simulink model "MEEN432_Project2_test"  (R2023b)
settings: Solver=VariableStepAuto  StartTime=0.0  StopTime=350  RelTol=1e-3
values from neighbouring files (symbols this model uses):
  alpha_max = 8 * pi/180    (= 0.13962634016)    [MEEN432_Project2_init.m]
  Calpha_f = 40000    [MEEN432_Project2_init.m]
  Calpha_r = 40000    [MEEN432_Project2_init.m]
  inertia = 1600    [MEEN432_Project2_init.m]
  lf = 1.5    [MEEN432_Project2_init.m]
  lr = 1.0    (= 1)    [MEEN432_Project2_init.m]
  mass = 1000    [MEEN432_Project2_init.m]
  omega0 = 0    [MEEN432_Project2_init.m]
  psi0 = 0    [MEEN432_Project2_init.m]
  vd = 10    [MEEN432_Project2_init.m]
  vx_max = 0.1    [MEEN432_Project2_init.m]
  vy0 = 0    [MEEN432_Project2_init.m]
  x_track = [x1 , R*cos(t1) + L , x2, R*cos(t2)]    [MEEN432_Project2_init.m]
  y_track = [y1, R*sin(t1) + R , y2 , R*sin(t2) + R]    [MEEN432_Project2_init.m]
settings Model: Creator=flare  LastModifiedBy=flare

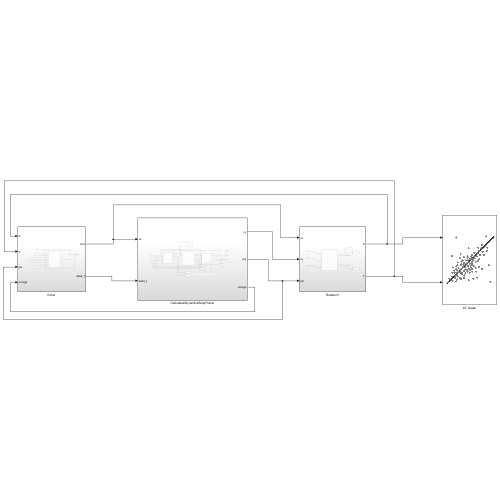
[thumbnail: Simulink's stored preview of the top-level diagram]
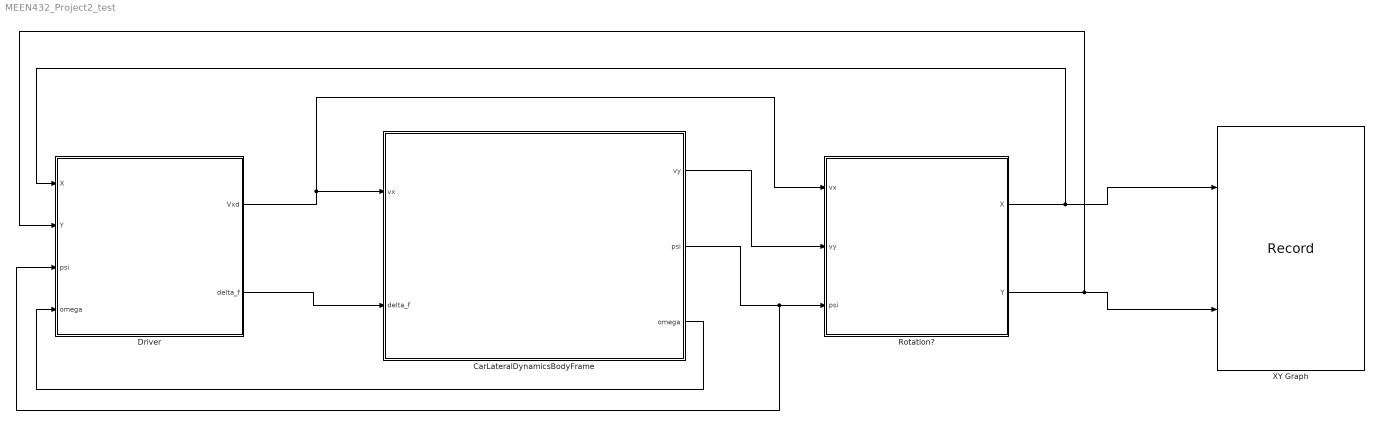
== system MEEN432_Project2_test ==
  CarLateralDynamicsBodyFrame : Subsystem
  Driver : Subsystem
  Rotation? : Subsystem
  XY Graph : Record  FileSettingsInternal="{\"entries\":[{\"content\":{\"excelSettings\":{\"content\":{},\"type\":\"Streamout.ExcelSettings\"}},\"type\":\"Streamout.FileSettingStorage\",\"uuid\":\"\"}],\"packageUris\":[\"http:\\/\\/schema.mathworks.com\\/mf0\\/streamout_blocks\\/R2020a\"],\"version\":\"1.0\"}"  Layout=[1 1]  SignalsInternal="{\"entries\":[{\"content\":{\"signals\":[{\"content\":{\"blockPath\":[],\"dimensions\":[1],\"domain\":\"\",\"lineColor\":\"#139fff\",\"plots\":[1],\"port\":1,\"sid\":[\"\"],\"signalID\":693,\"signalName\":\"Rotation?:1\"},\"type\":\"RecordBlkView.Signal\",\"uuid\":\"\"},{\"content\":{\"blockPath\":[],\"dimensions\":[1],\"domain\":\"\",\"lineColor\":\"#ff6929\",\"plots\":[1],\"port\":2,\"sid\":[\"\"],\"signalID\":697,\"signalName\":\"Rotation?:2\"},\"type\":\"RecordBlkView.Signal\",\"uuid\":\"\"}]},\"type\":\"RecordBlkView.InputSignals\",\"uuid\":\"\"}],\"packageUris\":[\"http:\\/\\/schema.mathworks.com\\/mf0\\/streamout_blocks\\/R2020a\"],\"version\":\"1.0\"}"  VisualizationBindings="{\"xyplotplugin\":{\"info\":[{\"series\":[{\"bindingParametersList\":[{\"parameter\":\"X-Axis\",\"signalID\":693,\"signalName\":\"Rotation?:1\"},{\"parameter\":\"Y-Axis\",\"signalID\":697,\"signalName\":\"Rotation?:2\"}],\"seriesID\":48390}],\"subplotID\":1}]}}"  CompatibilityTag=XY
  wires:
  Rotation?/1(X) -> Driver/1(X), XY Graph/1
  Rotation?/2(Y) -> Driver/2(Y), XY Graph/2
  Driver/1(Vxd) -> Rotation?/1(vx), CarLateralDynamicsBodyFrame/1(vx)
  Driver/2(delta_f) -> CarLateralDynamicsBodyFrame/2(delta_f)
  CarLateralDynamicsBodyFrame/1(vy) -> Rotation?/2(vy)
  CarLateralDynamicsBodyFrame/2(psi) -> Driver/3(psi), Rotation?/3(psi)
  CarLateralDynamicsBodyFrame/3(omega) -> Driver/4(omega)

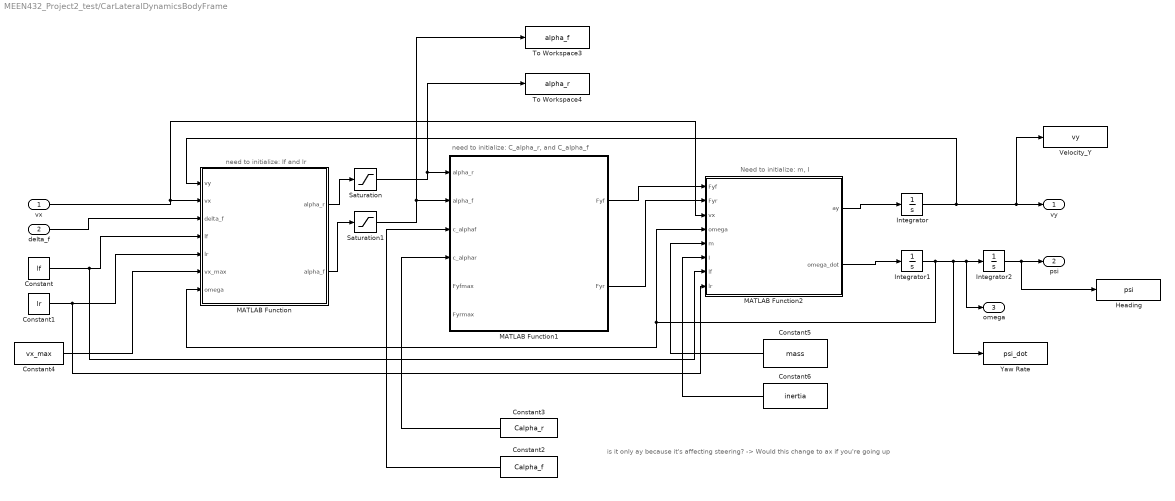
== system MEEN432_Project2_test/CarLateralDynamicsBodyFrame ==
  note: need to initialize: lf and lr
  note: need to initialize: C_alpha_r, and C_alpha_f
  note: is it only ay because it's affecting steering? -> Would this change to ax if you're going up
  note: Need to initialize: m, I
  vx : Inport
  delta_f : Inport  Port=2
  Constant : Constant  Value=lf
  Constant1 : Constant  Value=lr
  Constant2 : Constant  Value=Calpha_f
  Constant3 : Constant  Value=Calpha_r
  Constant4 : Constant  Value=vx_max
  Constant5 : Constant  Value=mass
  Constant6 : Constant  Value=inertia
  Heading : ToWorkspace  VariableName=psi  SaveFormat=Timeseries  SampleTime=-1
  Integrator : Integrator  InitialCondition=vy0
  Integrator1 : Integrator  InitialCondition=omega0
  Integrator2 : Integrator  InitialCondition=psi0
  MATLAB Function : MATLAB Function  TreatAsAtomicUnit=on
  MATLAB Function1 : MATLAB Function  TreatAsAtomicUnit=on
  MATLAB Function2 : MATLAB Function  TreatAsAtomicUnit=on
  Saturation : Saturate  UpperLimit=alpha_max
  Saturation1 : Saturate  UpperLimit=alpha_max
  To Workspace3 : ToWorkspace  VariableName=alpha_f  SaveFormat=Timeseries  SampleTime=-1
  To Workspace4 : ToWorkspace  VariableName=alpha_r  SaveFormat=Timeseries  SampleTime=-1
  Velocity_Y : ToWorkspace  VariableName=vy  SaveFormat=Timeseries  SampleTime=-1
  Yaw Rate : ToWorkspace  VariableName=psi_dot  SaveFormat=Timeseries  SampleTime=-1
  vy : Outport
  psi : Outport  Port=2
  omega : Outport  Port=3
  wires:
  MATLAB Function/1(alpha_r) -> Saturation/1
  MATLAB Function/2(alpha_f) -> Saturation1/1
  MATLAB Function2/2(omega_dot) -> Integrator1/1
  MATLAB Function2/1(ay) -> Integrator/1
  Integrator1/1 -> MATLAB Function2/4(omega), MATLAB Function/7(omega), Yaw Rate/1, omega/1, Integrator2/1
  Integrator/1 -> MATLAB Function/1(vy), Velocity_Y/1, vy/1
  Integrator2/1 -> Heading/1, psi/1
  vx/1 -> MATLAB Function2/3(vx), MATLAB Function/2(vx)
  delta_f/1 -> MATLAB Function/3(delta_f)
  Saturation/1 -> To Workspace4/1, MATLAB Function1/1(alpha_r)
  Saturation1/1 -> To Workspace3/1, MATLAB Function1/2(alpha_f)
  MATLAB Function1/1(Fyf) -> MATLAB Function2/1(Fyf)
  MATLAB Function1/2(Fyr) -> MATLAB Function2/2(Fyr)
  Constant/1 -> MATLAB Function2/7(lf), MATLAB Function/4(lf)
  Constant1/1 -> MATLAB Function2/8(lr), MATLAB Function/5(lr)
  Constant2/1 -> MATLAB Function1/3(c_alphaf)
  Constant3/1 -> MATLAB Function1/4(c_alphar)
  Constant4/1 -> MATLAB Function/6(vx_max)
  Constant5/1 -> MATLAB Function2/5(m)
  Constant6/1 -> MATLAB Function2/6(I)

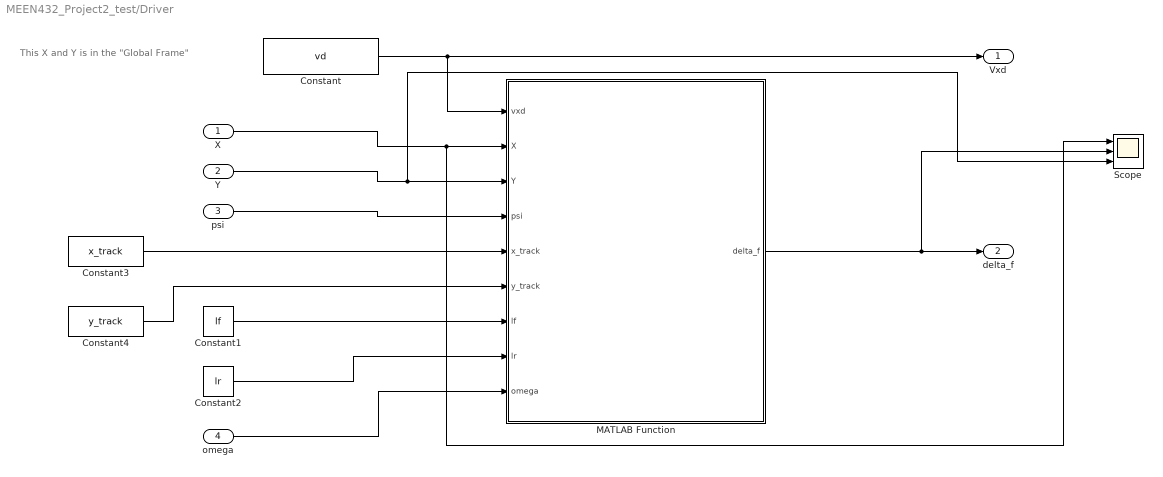
== system MEEN432_Project2_test/Driver ==
  note: This X and Y is in the "Global Frame"
  X : Inport
  Y : Inport  Port=2
  psi : Inport  Port=3
  omega : Inport  Port=4
  Constant : Constant  Value=vd
  Constant1 : Constant  Value=lf
  Constant2 : Constant  Value=lr
  Constant3 : Constant  Value=x_track  VectorParams1D=off
  Constant4 : Constant  Value=y_track  VectorParams1D=off
  MATLAB Function : MATLAB Function  TreatAsAtomicUnit=on
  Scope : Scope  NumInputPorts=3
  Vxd : Outport
  delta_f : Outport  Port=2
  wires:
  Y/1 -> Scope/3, MATLAB Function/3(Y)
  psi/1 -> MATLAB Function/4(psi)
  omega/1 -> MATLAB Function/9(omega)
  MATLAB Function/1(delta_f) -> Scope/2, delta_f/1
  X/1 -> Scope/1, MATLAB Function/2(X)
  Constant1/1 -> MATLAB Function/7(lf)
  Constant2/1 -> MATLAB Function/8(lr)
  Constant/1 -> MATLAB Function/1(vxd), Vxd/1
  Constant3/1 -> MATLAB Function/5(x_track)
  Constant4/1 -> MATLAB Function/6(y_track)

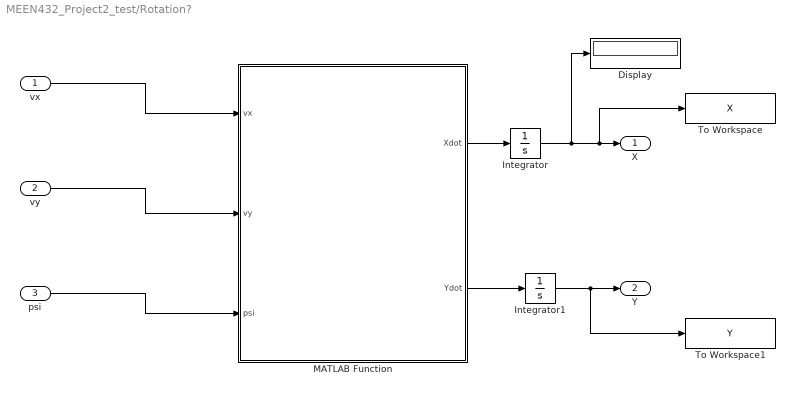
== system MEEN432_Project2_test/Rotation? ==
  vx : Inport
  vy : Inport  Port=2
  psi : Inport  Port=3
  Display : Display
  Integrator : Integrator
  Integrator1 : Integrator
  MATLAB Function : MATLAB Function  TreatAsAtomicUnit=on
  To Workspace : ToWorkspace  VariableName=X  SaveFormat=Timeseries  SampleTime=-1
  To Workspace1 : ToWorkspace  VariableName=Y  SaveFormat=Timeseries  SampleTime=-1
  X : Outport
  Y : Outport  Port=2
  wires:
  vx/1 -> MATLAB Function/1(vx)
  vy/1 -> MATLAB Function/2(vy)
  MATLAB Function/2(Ydot) -> Integrator1/1
  Integrator1/1 -> To Workspace1/1, Y/1
  psi/1 -> MATLAB Function/3(psi)
  MATLAB Function/1(Xdot) -> Integrator/1
  Integrator/1 -> Display/1, To Workspace/1, X/1

== matlab function MEEN432_Project2_test/CarLateralDynamicsBodyFrame/MATLAB Function ==
  data: vy input; alpha_r output; vx input; delta_f input; lf input; lr input; vx_max input; omega input; alpha_f output
function [alpha_r, alpha_f] = fcn(vy, vx, delta_f, lf, lr, vx_max, omega)

if abs(vx) > vx_max
    alpha_f = delta_f - atan((vy+lf*omega)/vx);
    alpha_r = atan((vy-lr*omega)/vx);
else
    alpha_f = 0;
    alpha_r = 0;
end

end

== matlab function MEEN432_Project2_test/Driver/MATLAB Function ==
  data: vxd input; X input; Y input; psi input; x_track input; y_track input; lf input; lr input; omega input; delta_f output
function delta_f = fcn(vxd, X, Y, psi, x_track, y_track, lf, lr, omega)

wheelBase = lr + lf;
point = [X,Y];
distance = [];
track = [x_track ; y_track];
for i = 1:length(track)
     distance(end+1) = ((track(1,i)-point(1))^2+(track(2,i)-point(2))^2)^(1/2);
end
[~,min_index] = min(distance);
k = min_index+10; %Going two point up the curve for a smoother turn
%To prevent out of bounds index
if(k>length(track))
    k = length(track);
end
target_point = track(:,k);

alpha = atan2(target_point(2)-point(2), target_point(1)-point(1))-psi;
psi_dot = 2*vxd*sin(alpha)/wheelBase;
delta_f = psi_dot-omega;

== matlab function MEEN432_Project2_test/CarLateralDynamicsBodyFrame/MATLAB Function1 ==
  data: alpha_r input; Fyf output; alpha_f input; Fyr output; c_alphaf input; c_alphar input; Fyfmax input; Fyrmax input
function [Fyf, Fyr] = fcn(alpha_r, alpha_f, c_alphaf, c_alphar, Fyfmax, Fyrmax)

%solve for Fyf and Fyr with given/solved values
yf = c_alphaf * alpha_r;
yr = c_alphar * alpha_f;

%check to make sure it's not past the max
Fyf = min(yf, Fyfmax);
Fyr = min(yr, Fyrmax);

== matlab function MEEN432_Project2_test/CarLateralDynamicsBodyFrame/MATLAB Function2 ==
  data: Fyf input; ay output; Fyr input; vx input; omega input; omega_dot output; m input; I input; lf input; lr input
function [ay, omega_dot] = fcn(Fyf, Fyr, vx, omega, m, I, lf, lr)

ay= -(vx*omega) + (Fyf+Fyr)/m;
omega_dot = (Fyf*lf - Fyr*lr)/I;

== matlab function MEEN432_Project2_test/Rotation?/MATLAB Function ==
  data: vx input; Xdot output; vy input; psi input; Ydot output
function [Xdot, Ydot] = fcn(vx, vy, psi)
    temp = TF(psi) * [vx;vy]; 
    Xdot = temp(1);
    Ydot = temp(2);
  
end

function y = TF(psi)
    y = [cos(psi), -sin(psi); sin(psi), cos(psi)];
end
